simulink model "SecRwLtStCalib"  (R2024b)
settings: Solver=FixedStepDiscrete  StartTime=0.0  StopTime=10.0  FixedStep=0.01  RelTol=1e-3
model workspace (MAT data in the model file):
  KeSMSwAcsMd6SecRwLtStBkReclnUpwdDnwdPos1Max_Val : Simulink.Parameter (value not decoded)
  KeSMSwAcsMd6SecRwLtStBkReclnUpwdDnwdPos1Min_Val : Simulink.Parameter (value not decoded)
  KeSMSwAcsMd6SecRwLtStBkReclnUpwdDnwdPos1_Val : Simulink.Parameter (value not decoded)
  KeSMSwAcsMd6SecRwLtStBkReclnUpwdDnwdPosMax_Val : Simulink.Parameter (value not decoded)
  KeSMSwAcsMd6SecRwLtStBkReclnUpwdDnwdPosMin_Val : Simulink.Parameter (value not decoded)
  KeSMSwAcsMd6SecRwLtStBkReclnUpwdDnwdPos_Val : Simulink.Parameter (value not decoded)
symbols that are objects in the model workspace (value not decoded): KeSMSwAcsMd6SecRwLtStBkReclnUpwdDnwdPos1_Val, KeSMSwAcsMd6SecRwLtStBkReclnUpwdDnwdPos1Max_Val, KeSMSwAcsMd6SecRwLtStBkReclnUpwdDnwdPos1Min_Val, KeSMSwAcsMd6SecRwLtStBkReclnUpwdDnwdPos_Val, KeSMSwAcsMd6SecRwLtStBkReclnUpwdDnwdPosMax_Val, KeSMSwAcsMd6SecRwLtStBkReclnUpwdDnwdPosMin_Val
undefined symbols (not defined in the file or in its folder): KeSMSw4SAcsMd21SecRwLtStBkReclnUpwdDnwdPos_Val, KeSMSw4SAcsMd21SecRwLtStBkReclnUpwdDnwdPosMax_Val, KeSMSw4SAcsMd21SecRwLtStBkReclnUpwdDnwdPosMin_Val, KeSMSw4SAcsMd21SecRwLtStFrwdBkwdPos_Val, KeSMSw4SAcsMd21SecRwLtStFrwdBkwdPosMax_Val, KeSMSw4SAcsMd21SecRwLtStFrwdBkwdPosMin_Val, KeSMSw4SAcsMd21SecRwLtStHdrstFrwdBkwdPos_Val, KeSMSw4SAcsMd21SecRwLtStHdrstFrwdBkwdPosMax_Val, KeSMSw4SAcsMd21SecRwLtStHdrstFrwdBkwdPosMin_Val, KeSMSw4SAcsMd21SecRwLtStHdrstUpwdDnwdPos_Val, KeSMSw4SAcsMd21SecRwLtStHdrstUpwdDnwdPosMax_Val, KeSMSw4SAcsMd21SecRwLtStHdrstUpwdDnwdPosMin_Val, KeSMSw4SAcsMd22SecRwLtStBkReclnUpwdDnwdPos1_Val, KeSMSw4SAcsMd22SecRwLtStBkReclnUpwdDnwdPos2_Val, KeSMSw4SAcsMd22SecRwLtStBkReclnUpwdDnwdPos2Max_Val, KeSMSw4SAcsMd22SecRwLtStBkReclnUpwdDnwdPos2Min_Val, KeSMSw4SAcsMd22SecRwLtStBkReclnUpwdDnwdPosMax_Val, KeSMSw4SAcsMd22SecRwLtStBkReclnUpwdDnwdPosMin_Val, KeSMSw4SAcsMd22SecRwLtStFrwdBkwdPos_Val, KeSMSw4SAcsMd22SecRwLtStFrwdBkwdPosMax_Val, KeSMSw4SAcsMd22SecRwLtStFrwdBkwdPosMin_Val, KeSMSw4SAcsMd22SecRwLtStFtrstUpwdDnwdPos_Val, KeSMSw4SAcsMd22SecRwLtStFtrstUpwdDnwdPosMax_Val, KeSMSw4SAcsMd22SecRwLtStFtrstUpwdDnwdPosMin_Val, KeSMSw4SAcsMd22SecRwLtStHdrstFrwdBkwdPos_Val, KeSMSw4SAcsMd22SecRwLtStHdrstFrwdBkwdPosMax_Val, KeSMSw4SAcsMd22SecRwLtStHdrstFrwdBkwdPosMin_Val, KeSMSw4SAcsMd22SecRwLtStHdrstUpwdDnwdPos_Val, KeSMSw4SAcsMd22SecRwLtStHdrstUpwdDnwdPosMax_Val, KeSMSw4SAcsMd22SecRwLtStHdrstUpwdDnwdPosMin_Val, KeSMSw4SAcsMd22SecRwLtStLegrstOtwdInwdPos_Val, KeSMSw4SAcsMd22SecRwLtStLegrstOtwdInwdPosMax_Val, KeSMSw4SAcsMd22SecRwLtStLegrstOtwdInwdPosMin_Val, KeSMSw4SAcsMd22SecRwLtStLegrstUpwdDnwdPos_Val, KeSMSw4SAcsMd22SecRwLtStLegrstUpwdDnwdPosMax_Val, KeSMSw4SAcsMd22SecRwLtStLegrstUpwdDnwdPosMin_Val, KeSMSw4SAcsMd25SecRwLtStBkReclnUpwdDnwdPos_Val, KeSMSw4SAcsMd25SecRwLtStBkReclnUpwdDnwdPosMax_Val, KeSMSw4SAcsMd25SecRwLtStBkReclnUpwdDnwdPosMin_Val, KeSMSw4SAcsMd25SecRwLtStFrwdBkwdPos_Val, KeSMSw4SAcsMd25SecRwLtStFrwdBkwdPosMax_Val, KeSMSw4SAcsMd25SecRwLtStFrwdBkwdPosMin_Val, KeSMSw4SAcsMd25SecRwLtStHdrstFrwdBkwdPos_Val, KeSMSw4SAcsMd25SecRwLtStHdrstFrwdBkwdPosMax_Val, KeSMSw4SAcsMd25SecRwLtStHdrstFrwdBkwdPosMin_Val, KeSMSw4SAcsMd25SecRwLtStHdrstUpwdDnwdPos_Val, KeSMSw4SAcsMd25SecRwLtStHdrstUpwdDnwdPosMax_Val, KeSMSw4SAcsMd25SecRwLtStHdrstUpwdDnwdPosMin_Val, KeSMSw4SAcsMd26SecRwLtStBkReclnUpwdDnwdPos_Val, KeSMSw4SAcsMd26SecRwLtStBkReclnUpwdDnwdPosMax_Val, KeSMSw4SAcsMd26SecRwLtStBkReclnUpwdDnwdPosMin_Val, KeSMSw4SAcsMd26SecRwLtStFrwdBkwdPos_Val, KeSMSw4SAcsMd26SecRwLtStFrwdBkwdPosMax_Val, KeSMSw4SAcsMd26SecRwLtStFrwdBkwdPosMin_Val, KeSMSw4SAcsMd26SecRwLtStFtrstUpwdDnwdPos_Val, KeSMSw4SAcsMd26SecRwLtStFtrstUpwdDnwdPosMax_Val, KeSMSw4SAcsMd26SecRwLtStFtrstUpwdDnwdPosMin_Val, KeSMSw4SAcsMd26SecRwLtStHdrstFrwdBkwdPos_Val, KeSMSw4SAcsMd26SecRwLtStHdrstFrwdBkwdPosMax_Val, KeSMSw4SAcsMd26SecRwLtStHdrstFrwdBkwdPosMin_Val ... (+496)
libraries: TrgtPosSelcLib x61, StIsPosChkLib x1, simulink x1
(part 6 of 8)

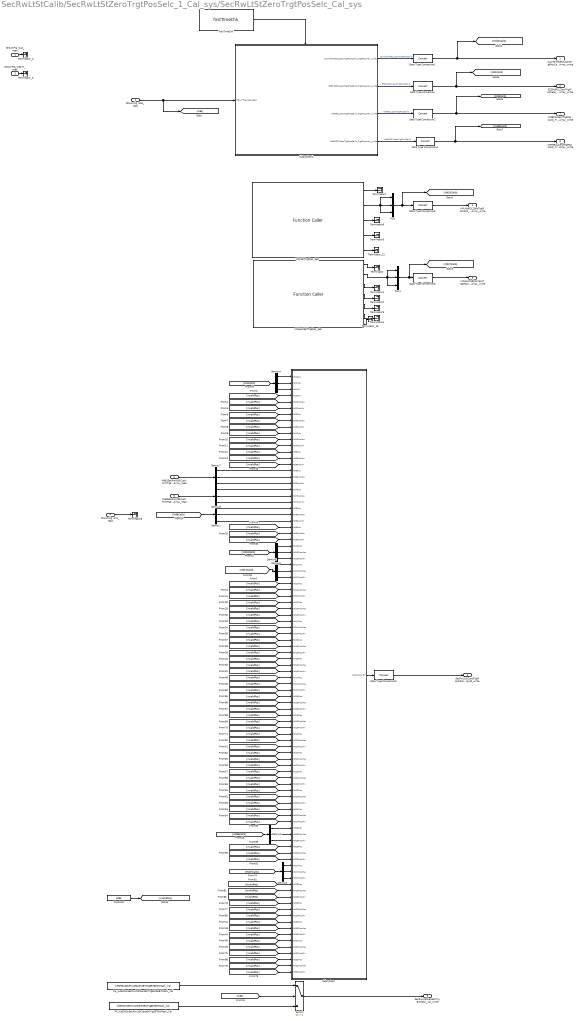
== system SecRwLtStCalib/SecRwLtStZeroTrgtPosSelc_1_Cal_sys/SecRwLtStZeroTrgtPosSelc_Cal_sys ==
  StNumFlg_Is4s_read : Inport
  StNumFlg_Is6s_read : Inport  Port=2
  StNumFlg_Is6s7s_read : Inport  Port=3
  StNumFlg_Is7s_read : Inport  Port=4
  Md61SecRwRtStCushFrntTrgtPosCalib_TrgtPosArray_read : Inport  Port=5
  Md62SecRwLtStCushFrntTrgtPosCalib_TrgtPosArray_read : Inport  Port=6
  Constant : Constant  Value=4095  OutDataTypeStr=uint16
  Data Type Conversion{,1..6} (7 alike) : DataTypeConversion  SaturateOnIntegerOverflow=off  RndMeth=Floor
  Demux{1..8} (8 alike) : Demux  Outputs=3
  Mux : Mux  Inputs=3
  Mux1 : Mux  Inputs=3
  PA_KeSMSwSecRwLtStZeroEnTrig5576sBitMask_Val : Constant  Value=KeSMSwSecRwLtStZeroEnTrig5576sBitMask_Val
  PA_KeSMSwSecRwLtStZeroEnTrig557BitMask_Val : Constant  Value=KeSMSwSecRwLtStZeroEnTrig557BitMask_Val
  Subsystem : Subsystem
  Subsystem1 : Subsystem
  Switch : Switch  Criteria=u2 > Threshold  SaturateOnIntegerOverflow=off  InputSameDT=off
  Terminator{,1..8} (9 alike) : Terminator
  Terminator_{3,5,12..13} (4 alike) : Terminator
  VIPL557TrgtPos_Get : FunctionCaller  FunctionPrototype=[SecRwLtStBkReclnTrgtPos,SecRwLtStZeroTrgtPos,SecRwLtStLgrstUpwdDnwdTrgtPos,SecRwLtStLgrstInwdOtwdTrgtPos,SecRwLtStFwdBkwdTrgtPos] = VIPL557TrgtPos_Get()  InputArgumentSpecifications=<Enter example>  OutputArgumentSpecifications=uint16(1), uint16(1), uint16(1), uint16(1), uint16(1)
  VIPLExit557TrgtPos_Get : FunctionCaller  FunctionPrototype=[SecRwLtStBkReclnTrgtPos,SecRwLtStZeroTrgtPos,SecRwLtStLgrstUpwdDnwdTrgtPos,SecRwLtStLgrstInwdOtwdTrgtPos,ThdRwLtStBkReclnTrgtPos,ThdRwLtStFwdBkwdTrgtPos,SecRwLtStFwdBkwdTrgtPos] = VIPLExit557TrgtPos_Get()  InputArgumentSpecifications=<Enter example>  OutputArgumentSpecifications=uint16(1), uint16(1), uint16(1), uint16(1), uint16(1), uint16(1), uint16(1)
  firstTimeChk : TrgtPosSelcLib/firstTimeChk  SystemSampleTime=-1  VariantActivationTime=update diagram  AllowFlexibleInterface=on  Latency=0  AutoFrameSizeCalculation=off
  ComfortMdR2LZeroTrgtPosCalib_TrgtPosArray_write : Outport  VectorParamsAs1DForOutWhenUnconnected=off
      settings: EnsureOutportIsVirtual=on
  EZEMdR2LZeroTrgtPosCalib_TrgtPosArray_write : Outport  Port=2  VectorParamsAs1DForOutWhenUnconnected=off
      settings: EnsureOutportIsVirtual=on
  SecRwLtStZeroTrgtPosCalibArray32_TrgtPosArray32_write : Outport  Port=3  VectorParamsAs1DForOutWhenUnconnected=off
      settings: EnsureOutportIsVirtual=on
  VIPLMdR2LZeroTrgtPosCalib_TrgtPosArray_write : Outport  Port=4  VectorParamsAs1DForOutWhenUnconnected=off
      settings: EnsureOutportIsVirtual=on
  VIPLExitMdR2LZeroTrgtPosCalib_TrgtPosArray_write : Outport  Port=5  VectorParamsAs1DForOutWhenUnconnected=off
      settings: EnsureOutportIsVirtual=on
  SecRwLtStZeroEnTrigBitMask_Val_write : Outport  Port=6  VectorParamsAs1DForOutWhenUnconnected=off
      settings: EnsureOutportIsVirtual=on
  Md8R2LZeroTrgtPosCalib_TrgtPosArray_write : Outport  Port=7  VectorParamsAs1DForOutWhenUnconnected=off
      settings: EnsureOutportIsVirtual=on
  Md56R2LZeroTrgtPosCalib_TrgtPosArray_write : Outport  Port=8  VectorParamsAs1DForOutWhenUnconnected=off
      settings: EnsureOutportIsVirtual=on
  wires:
  StNumFlg_Is4s_read/1 -> Terminator_3/1
  StNumFlg_Is6s7s_read/1 -> Terminator_5/1
  Mux/1 -> [Md10Calib], Data Type Conversion5/1
  VIPLExit557TrgtPos_Get/2 -> Mux1/3, Mux1/1, Mux1/2
  Mux1/1 -> [Md27Calib], Data Type Conversion6/1
  VIPLExit557TrgtPos_Get/1 -> Terminator/1
  VIPLExit557TrgtPos_Get/3 -> Terminator1/1
  VIPLExit557TrgtPos_Get/4 -> Terminator2/1
  VIPLExit557TrgtPos_Get/5 -> Terminator3/1
  VIPLExit557TrgtPos_Get/6 -> Terminator4/1
  VIPL557TrgtPos_Get/4 -> Terminator5/1
  VIPL557TrgtPos_Get/3 -> Terminator6/1
  VIPL557TrgtPos_Get/1 -> Terminator7/1
  VIPL557TrgtPos_Get/2 -> Mux/3, Mux/1, Mux/2
  Data Type Conversion3/1 -> SecRwLtStZeroTrgtPosCalibArray32_TrgtPosArray32_write/1
  Demux1/3 -> Subsystem/24(Md8PosMin)
  [invalidPos] -> Subsystem/85(Md29Pos)
  [invalidPos] -> Subsystem/10(Md4Pos)
  [invalidPos] -> Subsystem/50(Md17PosMax)
  [invalidPos] -> Subsystem/77(Md26PosMax)
  Demux1/1 -> Subsystem/22(Md8Pos)
  [invalidPos] -> Subsystem/9(Md3PosMin)
  [invalidPos] -> Subsystem/76(Md26Pos)
  [invalidPos] -> Subsystem/25(Md9Pos)
  [invalidPos] -> Subsystem/46(Md16Pos)
  [invalidPos] -> Subsystem/72(Md24PosMin)
  Demux5/3 -> Subsystem/30(Md10PosMin)
  [invalidPos] -> Subsystem/45(Md15PosMin)
  [invalidPos] -> Subsystem/63(Md21PosMin)
  [invalidPos] -> Subsystem/58(Md20Pos)
  [invalidPos] -> Subsystem/53(Md18PosMax)
  Demux4/1 -> Subsystem/1(Md1Pos)
  [invalidPos] -> Subsystem/55(Md19Pos)
  [invalidPos] -> Subsystem/86(Md29PosMax)
  [invalidPos] -> Subsystem/68(Md23PosMax)
  [invalidPos] -> Subsystem/62(Md21PosMax)
  [invalidPos] -> Subsystem/14(Md5PosMax)
  [invalidPos] -> Subsystem/87(Md29PosMin)
  Demux1/2 -> Subsystem/23(Md8PosMax)
  [invalidPos] -> Subsystem/26(Md9PosMax)
  [invalidPos] -> Subsystem/94(Md32Pos)
  [invalidPos] -> Subsystem/54(Md18PosMin)
  [invalidPos] -> Subsystem/61(Md21Pos)
  [invalidPos] -> Subsystem/5(Md2PosMax)
  [invalidPos] -> Subsystem/13(Md5Pos)
  [invalidPos] -> Subsystem/96(Md32PosMin)
  [invalidPos] -> Subsystem/59(Md20PosMax)
  [invalidPos] -> Subsystem/78(Md26PosMin)
  [invalidPos] -> Subsystem/11(Md4PosMax)
  Demux3/1 -> Subsystem/73(Md25Pos)
  [invalidPos] -> Subsystem/66(Md22PosMin)
  Demux4/2 -> Subsystem/2(Md1Max)
  [invalidPos] -> Subsystem/70(Md24Pos)
  [invalidPos] -> Subsystem/44(Md15PosMax)
  [invalidPos] -> Subsystem/60(Md20PosMin)
  [invalidPos] -> Subsystem/64(Md22Pos)
  [invalidPos] -> Subsystem/51(Md17PosMin)
  [invalidPos] -> Subsystem/43(Md15Pos)
  [invalidPos] -> Subsystem/57(Md19PosMin)
  [invalidPos] -> Subsystem/67(Md23Pos)
  [invalidPos] -> Subsystem/4(Md2Pos)
  [invalidPos] -> Subsystem/49(Md17Pos)
  [invalidPos] -> Subsystem/71(Md24PosMax)
  [invalidPos] -> Subsystem/65(Md22PosMax)
  [invalidPos] -> Subsystem/6(Md2PosMin)
  Demux3/3 -> Subsystem/75(Md25PosMin)
  [invalidPos] -> Subsystem/37(Md13Pos)
  [invalidPos] -> Subsystem/52(Md18Pos)
  Demux3/2 -> Subsystem/74(Md25PosMax)
  [invalidPos] -> Subsystem/27(Md9PosMin)
  [invalidPos] -> Subsystem/48(Md16PosMin)
  [invalidPos] -> Subsystem/41(Md14PosMax)
  Demux5/1 -> Subsystem/28(Md10Pos)
  [invalidPos] -> Subsystem/38(Md13PosMax)
  [invalidPos] -> Subsystem/47(Md16PosMax)
  [invalidPos] -> Subsystem/56(Md19PosMax)
  [invalidPos] -> Subsystem/39(Md13PosMin)
  [invalidPos] -> Subsystem/40(Md14Pos)
  Subsystem/1(CalibArray32) -> Data Type Conversion3/1
  [invalidPos] -> Subsystem/42(Md14PosMin)
  [invalidPos] -> Subsystem/12(Md4PosMin)
  [invalidPos] -> Subsystem/69(Md23PosMin)
  [invalidPos] -> Subsystem/82(Md28Pos)
  [invalidPos] -> Subsystem/15(Md5PosMin)
  Demux4/3 -> Subsystem/3(Md1Min)
  [invalidPos] -> Subsystem/95(Md32PosMax)
  [invalidPos] -> Subsystem/8(Md3PosMax)
  [invalidPos] -> Subsystem/7(Md3Pos)
  Demux5/2 -> Subsystem/29(Md10PosMax)
  [Md1Calib] -> Demux4/1
  [Md10Calib] -> Demux5/1
  Demux6/1 -> Subsystem/31(Md11Pos)
  Demux6/2 -> Subsystem/32(Md11PosMax)
  Demux6/3 -> Subsystem/33(Md11PosMin)
  [Md11Calib] -> Demux6/1
  [invalidPos] -> Subsystem/34(Md12Pos)
  [invalidPos] -> Subsystem/35(Md12PosMax)
  [invalidPos] -> Subsystem/36(Md12PosMin)
  [Md27Calib] -> Demux2/1
  Demux2/1 -> Subsystem/79(Md27Pos)
  Demux2/2 -> Subsystem/80(Md27PosMax)
  Demux2/3 -> Subsystem/81(Md27PosMin)
  [invalidPos] -> Subsystem/83(Md28PosMax)
  [invalidPos] -> Subsystem/84(Md28PosMin)
  [invalidPos] -> Subsystem/88(Md30Pos)
  [invalidPos] -> Subsystem/89(Md30PosMax)
  [invalidPos] -> Subsystem/90(Md30PosMin)
  [invalidPos] -> Subsystem/91(Md31Pos)
  [invalidPos] -> Subsystem/92(Md31PosMax)
  [invalidPos] -> Subsystem/93(Md31PosMin)
  Constant/1 -> [invalidPos]
  VIPL557TrgtPos_Get/5 -> Terminator_12/1
  VIPLExit557TrgtPos_Get/7 -> Terminator_13/1
  [Md8Calib] -> Demux1/1
  StNumFlg_Is7s_read/1 -> Terminator8/1
  Switch/1 -> SecRwLtStZeroEnTrigBitMask_Val_write/1
  [Is6s] -> Switch/2
  PA_KeSMSwSecRwLtStZeroEnTrig5576sBitMask_Val/1 -> Switch/1
  PA_KeSMSwSecRwLtStZeroEnTrig557BitMask_Val/1 -> Switch/3
  firstTimeChk/1 -> Subsystem1/Enable
  StNumFlg_Is6s_read/1 -> [Is6s], Subsystem1/1(StNumFlg_Is6s_read)
  Subsystem1/4(Md56R2LZeroTrgtPosCalib_TrgtPosArray_write) -> Data Type Conversion4/1  "Md56R2LZeroTrgtPosCalib"
  Subsystem1/1(ComfortMdR2LZeroTrgtPosCalib_TrgtPosArray_write) -> Data Type Conversion1/1  "ComfortMdR2LZeroTrgtPosCalib"
  Subsystem1/2(EZEMdR2LZeroTrgtPosCalib_TrgtPosArray_write) -> Data Type Conversion/1  "EZEMdR2LZeroTrgtPosCalib"
  Subsystem1/3(Md8R2LZeroTrgtPosCalib_TrgtPosArray_write) -> Data Type Conversion2/1  "Md8R2LZeroTrgtPosCalib"
  [Md56Calib] -> Demux3/1
  Data Type Conversion1/1 -> [Md11Calib], ComfortMdR2LZeroTrgtPosCalib_TrgtPosArray_write/1
  Data Type Conversion/1 -> [Md1Calib], EZEMdR2LZeroTrgtPosCalib_TrgtPosArray_write/1
  Data Type Conversion2/1 -> [Md8Calib], Md8R2LZeroTrgtPosCalib_TrgtPosArray_write/1
  Data Type Conversion4/1 -> [Md56Calib], Md56R2LZeroTrgtPosCalib_TrgtPosArray_write/1
  Data Type Conversion5/1 -> VIPLMdR2LZeroTrgtPosCalib_TrgtPosArray_write/1
  Data Type Conversion6/1 -> VIPLExitMdR2LZeroTrgtPosCalib_TrgtPosArray_write/1
  Demux7/1 -> Subsystem/16(Md6Pos)
  Demux7/2 -> Subsystem/17(Md6PosMax)
  Demux7/3 -> Subsystem/18(Md6PosMin)
  Md61SecRwRtStCushFrntTrgtPosCalib_TrgtPosArray_read/1 -> Demux7/1
  Demux8/1 -> Subsystem/19(Md7Pos)
  Demux8/2 -> Subsystem/20(Md7PosMax)
  Demux8/3 -> Subsystem/21(Md7PosMin)
  Md62SecRwLtStCushFrntTrgtPosCalib_TrgtPosArray_read/1 -> Demux8/1

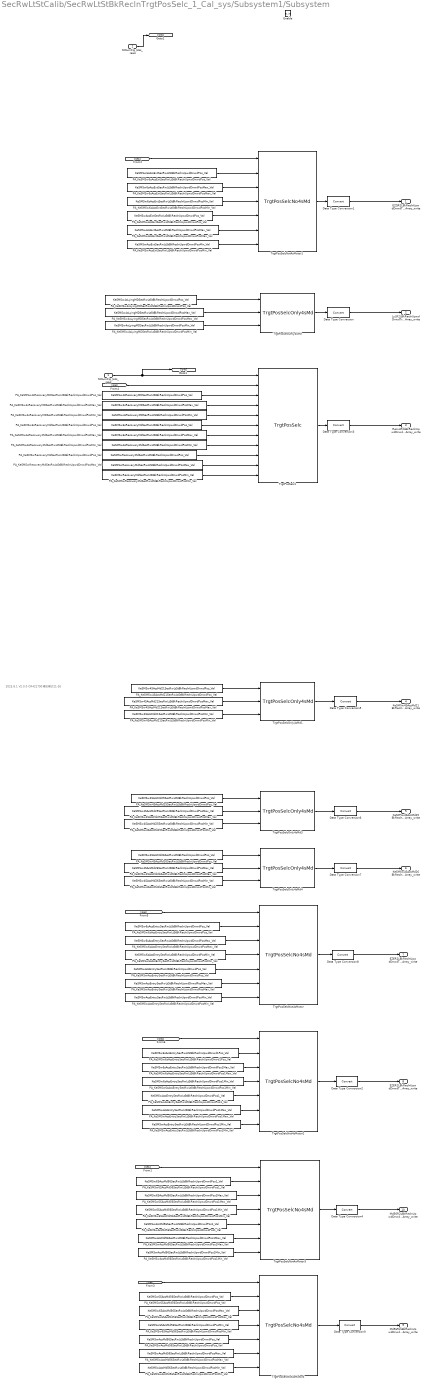
== system SecRwLtStCalib/SecRwLtStBkReclnTrgtPosSelc_1_Cal_sys/Subsystem1/Subsystem ==
  note: 2023.8.1 V2.0.0 CR421790 增加模式21-26
  StNumFlg_Is4s_read : Inport
  StNumFlg_Is6s_read : Inport  Port=2
  Enable : EnablePort
  Data Type Conversion{,1..9} (10 alike) : DataTypeConversion  SaturateOnIntegerOverflow=off  RndMeth=Floor
  PA_KeSMSw4SAcsMd21SecRwLtStBkReclnUpwdDnwdPosMax_Val : Constant  Value=KeSMSw4SAcsMd21SecRwLtStBkReclnUpwdDnwdPosMax_Val
  PA_KeSMSw4SAcsMd21SecRwLtStBkReclnUpwdDnwdPosMin_Val : Constant  Value=KeSMSw4SAcsMd21SecRwLtStBkReclnUpwdDnwdPosMin_Val
  PA_KeSMSw4SAcsMd21SecRwLtStBkReclnUpwdDnwdPos_Val : Constant  Value=KeSMSw4SAcsMd21SecRwLtStBkReclnUpwdDnwdPos_Val
  PA_KeSMSw4SAcsMd25SecRwLtStBkReclnUpwdDnwdPosMax_Val : Constant  Value=KeSMSw4SAcsMd25SecRwLtStBkReclnUpwdDnwdPosMax_Val
  PA_KeSMSw4SAcsMd25SecRwLtStBkReclnUpwdDnwdPosMin_Val : Constant  Value=KeSMSw4SAcsMd25SecRwLtStBkReclnUpwdDnwdPosMin_Val
  PA_KeSMSw4SAcsMd25SecRwLtStBkReclnUpwdDnwdPos_Val : Constant  Value=KeSMSw4SAcsMd25SecRwLtStBkReclnUpwdDnwdPos_Val
  PA_KeSMSw4SAcsMd26SecRwLtStBkReclnUpwdDnwdPosMax_Val : Constant  Value=KeSMSw4SAcsMd26SecRwLtStBkReclnUpwdDnwdPosMax_Val
  PA_KeSMSw4SAcsMd26SecRwLtStBkReclnUpwdDnwdPosMin_Val : Constant  Value=KeSMSw4SAcsMd26SecRwLtStBkReclnUpwdDnwdPosMin_Val
  PA_KeSMSw4SAcsMd26SecRwLtStBkReclnUpwdDnwdPos_Val : Constant  Value=KeSMSw4SAcsMd26SecRwLtStBkReclnUpwdDnwdPos_Val
  PA_KeSMSw4sLyingMDSecRwLtStBkReclnUpwdDnwdPosMax_Val : Constant  Value=KeSMSw4sLyingMDSecRwLtStBkReclnUpwdDnwdPosMax_Val
  PA_KeSMSw4sLyingMDSecRwLtStBkReclnUpwdDnwdPosMin_Val : Constant  Value=KeSMSw4sLyingMDSecRwLtStBkReclnUpwdDnwdPosMin_Val
  PA_KeSMSw4sLyingMDSecRwLtStBkReclnUpwdDnwdPos_Val : Constant  Value=KeSMSw4sLyingMDSecRwLtStBkReclnUpwdDnwdPos_Val
  PA_KeSMSw4sRecoveryMDSecRwLtStBkReclnUpwdDnwdPosMax_Val : Constant  Value=KeSMSw4sRecoveryMDSecRwLtStBkReclnUpwdDnwdPosMax_Val
  PA_KeSMSw4sRecoveryMDSecRwLtStBkReclnUpwdDnwdPosMin_Val : Constant  Value=KeSMSw4sRecoveryMDSecRwLtStBkReclnUpwdDnwdPosMin_Val
  PA_KeSMSw4sRecoveryMDSecRwLtStBkReclnUpwdDnwdPos_Val : Constant  Value=KeSMSw4sRecoveryMDSecRwLtStBkReclnUpwdDnwdPos_Val
  PA_KeSMSw6SAcsMd56SecRwLtStBkReclnUpwdDnwdPos1Max_Val : Constant  Value=KeSMSw6SAcsMd56SecRwLtStBkReclnUpwdDnwdPos1Max_Val
  PA_KeSMSw6SAcsMd56SecRwLtStBkReclnUpwdDnwdPos1Min_Val : Constant  Value=KeSMSw6SAcsMd56SecRwLtStBkReclnUpwdDnwdPos1Min_Val
  PA_KeSMSw6SAcsMd56SecRwLtStBkReclnUpwdDnwdPos1_Val : Constant  Value=KeSMSw6SAcsMd56SecRwLtStBkReclnUpwdDnwdPos1_Val
  PA_KeSMSw6SAcsMd56SecRwLtStBkReclnUpwdDnwdPosMax_Val : Constant  Value=KeSMSw6SAcsMd56SecRwLtStBkReclnUpwdDnwdPosMax_Val
  PA_KeSMSw6SAcsMd56SecRwLtStBkReclnUpwdDnwdPosMin_Val : Constant  Value=KeSMSw6SAcsMd56SecRwLtStBkReclnUpwdDnwdPosMin_Val
  PA_KeSMSw6SAcsMd56SecRwLtStBkReclnUpwdDnwdPos_Val : Constant  Value=KeSMSw6SAcsMd56SecRwLtStBkReclnUpwdDnwdPos_Val
  PA_KeSMSw6sAcsEntrySecRwLtStBkReclnUpwdDnwd1Pos_Val : Constant  Value=KeSMSw6sAcsEntrySecRwLtStBkReclnUpwdDnwd1Pos_Val
  PA_KeSMSw6sAcsEntrySecRwLtStBkReclnUpwdDnwdPos1Max_Val : Constant  Value=KeSMSw6sAcsEntrySecRwLtStBkReclnUpwdDnwdPos1Max_Val
  PA_KeSMSw6sAcsEntrySecRwLtStBkReclnUpwdDnwdPos1Min_Val : Constant  Value=KeSMSw6sAcsEntrySecRwLtStBkReclnUpwdDnwdPos1Min_Val
  PA_KeSMSw6sAcsEntrySecRwLtStBkReclnUpwdDnwdPosMax_Val : Constant  Value=KeSMSw6sAcsEntrySecRwLtStBkReclnUpwdDnwdPosMax_Val
  PA_KeSMSw6sAcsEntrySecRwLtStBkReclnUpwdDnwdPosMin_Val : Constant  Value=KeSMSw6sAcsEntrySecRwLtStBkReclnUpwdDnwdPosMin_Val
  PA_KeSMSw6sAcsEntrySecRwLtStBkReclnUpwdDnwdPos_Val : Constant  Value=KeSMSw6sAcsEntrySecRwLtStBkReclnUpwdDnwdPos_Val
  PA_KeSMSw6sAcsExtSecRwLtStBkReclnUpwdDnwdPosMax_Val : Constant  Value=KeSMSw6sAcsExtSecRwLtStBkReclnUpwdDnwdPosMax_Val
  PA_KeSMSw6sAcsExtSecRwLtStBkReclnUpwdDnwdPosMin_Val : Constant  Value=KeSMSw6sAcsExtSecRwLtStBkReclnUpwdDnwdPosMin_Val
  PA_KeSMSw6sAcsExtSecRwLtStBkReclnUpwdDnwdPos_Val : Constant  Value=KeSMSw6sAcsExtSecRwLtStBkReclnUpwdDnwdPos_Val
  PA_KeSMSw6sRecoveryMdSecRwLtStBkReclnUpwdDnwdPosMax_Val : Constant  Value=KeSMSw6sRecoveryMdSecRwLtStBkReclnUpwdDnwdPosMax_Val
  PA_KeSMSw6sRecoveryMdSecRwLtStBkReclnUpwdDnwdPosMin_Val : Constant  Value=KeSMSw6sRecoveryMdSecRwLtStBkReclnUpwdDnwdPosMin_Val
  PA_KeSMSw6sRecoveryMdSecRwLtStBkReclnUpwdDnwdPos_Val : Constant  Value=KeSMSw6sRecoveryMdSecRwLtStBkReclnUpwdDnwdPos_Val
  PA_KeSMSwAcsEntrySecRwLtStBkReclnUpwdDnwdPos1Max_Val : Constant  Value=KeSMSwAcsEntrySecRwLtStBkReclnUpwdDnwdPos1Max_Val
  PA_KeSMSwAcsEntrySecRwLtStBkReclnUpwdDnwdPos1Min_Val : Constant  Value=KeSMSwAcsEntrySecRwLtStBkReclnUpwdDnwdPos1Min_Val
  PA_KeSMSwAcsEntrySecRwLtStBkReclnUpwdDnwdPos1_Val : Constant  Value=KeSMSwAcsEntrySecRwLtStBkReclnUpwdDnwdPos1_Val
  PA_KeSMSwAcsEntrySecRwLtStBkReclnUpwdDnwdPosMax_Val : Constant  Value=KeSMSwAcsEntrySecRwLtStBkReclnUpwdDnwdPosMax_Val
  PA_KeSMSwAcsEntrySecRwLtStBkReclnUpwdDnwdPosMin_Val : Constant  Value=KeSMSwAcsEntrySecRwLtStBkReclnUpwdDnwdPosMin_Val
  PA_KeSMSwAcsEntrySecRwLtStBkReclnUpwdDnwdPos_Val : Constant  Value=KeSMSwAcsEntrySecRwLtStBkReclnUpwdDnwdPos_Val
  PA_KeSMSwAcsExtSecRwLtStBkReclnUpwdDnwdPosMax_Val : Constant  Value=KeSMSwAcsExtSecRwLtStBkReclnUpwdDnwdPosMax_Val
  PA_KeSMSwAcsExtSecRwLtStBkReclnUpwdDnwdPosMin_Val : Constant  Value=KeSMSwAcsExtSecRwLtStBkReclnUpwdDnwdPosMin_Val
  PA_KeSMSwAcsExtSecRwLtStBkReclnUpwdDnwdPos_Val : Constant  Value=KeSMSwAcsExtSecRwLtStBkReclnUpwdDnwdPos_Val
  PA_KeSMSwAcsMd56SecRwLtStBkReclnUpwdDnwdPos1Max_Val : Constant  Value=KeSMSwAcsMd56SecRwLtStBkReclnUpwdDnwdPos1Max_Val
  PA_KeSMSwAcsMd56SecRwLtStBkReclnUpwdDnwdPos1Min_Val : Constant  Value=KeSMSwAcsMd56SecRwLtStBkReclnUpwdDnwdPos1Min_Val
  PA_KeSMSwAcsMd56SecRwLtStBkReclnUpwdDnwdPos1_Val : Constant  Value=KeSMSwAcsMd56SecRwLtStBkReclnUpwdDnwdPos1_Val
  PA_KeSMSwAcsMd56SecRwLtStBkReclnUpwdDnwdPosMax_Val : Constant  Value=KeSMSwAcsMd56SecRwLtStBkReclnUpwdDnwdPosMax_Val
  PA_KeSMSwAcsMd56SecRwLtStBkReclnUpwdDnwdPosMin_Val : Constant  Value=KeSMSwAcsMd56SecRwLtStBkReclnUpwdDnwdPosMin_Val
  PA_KeSMSwAcsMd56SecRwLtStBkReclnUpwdDnwdPos_Val : Constant  Value=KeSMSwAcsMd56SecRwLtStBkReclnUpwdDnwdPos_Val
  PA_KeSMSwRecoveryMdSecRwLtStBkReclnUpwdDnwdPosMax_Val : Constant  Value=KeSMSwRecoveryMdSecRwLtStBkReclnUpwdDnwdPosMax_Val
  PA_KeSMSwRecoveryMdSecRwLtStBkReclnUpwdDnwdPosMin_Val : Constant  Value=KeSMSwRecoveryMdSecRwLtStBkReclnUpwdDnwdPosMin_Val
  PA_KeSMSwRecoveryMdSecRwLtStBkReclnUpwdDnwdPos_Val : Constant  Value=KeSMSwRecoveryMdSecRwLtStBkReclnUpwdDnwdPos_Val
  TrgtPosSelc1 : TrgtPosSelcLib/TrgtPosSelc  SystemSampleTime=-1  VariantActivationTime=update diagram  AllowFlexibleInterface=on  Latency=0  AutoFrameSizeCalculation=off
  TrgtPosSelcNot4sMotor{,1..4} (5 alike) : TrgtPosSelcLib/TrgtPosSelcNo4sMd  SystemSampleTime=-1  VariantActivationTime=update diagram  AllowFlexibleInterface=on  Latency=0  AutoFrameSizeCalculation=off
  TrgtPosSelcOnly4sMd{,1,3..4} (4 alike) : TrgtPosSelcLib/TrgtPosSelcOnly4sMd  SystemSampleTime=-1  VariantActivationTime=update diagram  AllowFlexibleInterface=on  Latency=0  AutoFrameSizeCalculation=off
  EZQR2LBkReclnUpwdDnwdTrgtPosCalib_TrgtPosArray_write : Outport  VectorParamsAs1DForOutWhenUnconnected=off
      settings: EnsureOutportIsVirtual=on
  LyLR2LBkReclnUpwdDnwdTrgtPosCalib_TrgtPosArray_write : Outport  Port=2  VectorParamsAs1DForOutWhenUnconnected=off
  RecvLR2LBkReclnUpwdDnwdTrgtPosCalib_TrgtPosArray_write : Outport  Port=3  VectorParamsAs1DForOutWhenUnconnected=off
      settings: EnsureOutportIsVirtual=on
  KeSMSw4SAcsMd21BkReclnUpwdDnwdTrgtPosCalib_TrgtPosArray_write : Outport  Port=4  InitialOutput=0  VectorParamsAs1DForOutWhenUnconnected=off
  KeSMSw4SAcsMd25BkReclnUpwdDnwdTrgtPosCalib_TrgtPosArray_write : Outport  Port=5  InitialOutput=0  VectorParamsAs1DForOutWhenUnconnected=off
  KeSMSw4SAcsMd26BkReclnUpwdDnwdTrgtPosCalib_TrgtPosArray_write : Outport  Port=6  InitialOutput=0  VectorParamsAs1DForOutWhenUnconnected=off
  EZER2LBkReclnUpwdDnwdTrgtPosCalib_TrgtPosArray_write : Outport  Port=7  VectorParamsAs1DForOutWhenUnconnected=off
  EZER2LBkReclnUpwdDnwdTrgtPosCalib1_TrgtPosArray_write : Outport  Port=8  VectorParamsAs1DForOutWhenUnconnected=off
  Md56R2LBkReclnUpwdDnwdTrgtPosCalib_TrgtPosArray_write : Outport  Port=9  VectorParamsAs1DForOutWhenUnconnected=off
      settings: EnsureOutportIsVirtual=on
  Md56R2LBkReclnUpwdDnwdTrgtPosCalib1_TrgtPosArray_write : Outport  Port=10  VectorParamsAs1DForOutWhenUnconnected=off
      settings: EnsureOutportIsVirtual=on
  wires:
  [is6s] -> TrgtPosSelcNot4sMotor1/1
  PA_KeSMSw4sLyingMDSecRwLtStBkReclnUpwdDnwdPosMax_Val/1 -> TrgtPosSelcOnly4sMd/2
  PA_KeSMSwAcsExtSecRwLtStBkReclnUpwdDnwdPosMin_Val/1 -> TrgtPosSelcNot4sMotor1/7
  PA_KeSMSw4sLyingMDSecRwLtStBkReclnUpwdDnwdPos_Val/1 -> TrgtPosSelcOnly4sMd/1
  TrgtPosSelcOnly4sMd/1 -> Data Type Conversion/1
  StNumFlg_Is4s_read/1 -> [is4s], TrgtPosSelc1/1
  PA_KeSMSw6sAcsExtSecRwLtStBkReclnUpwdDnwdPos_Val/1 -> TrgtPosSelcNot4sMotor1/2
  PA_KeSMSw4sRecoveryMDSecRwLtStBkReclnUpwdDnwdPosMax_Val/1 -> TrgtPosSelc1/4
  PA_KeSMSw4sLyingMDSecRwLtStBkReclnUpwdDnwdPosMin_Val/1 -> TrgtPosSelcOnly4sMd/3
  PA_KeSMSw4sRecoveryMDSecRwLtStBkReclnUpwdDnwdPos_Val/1 -> TrgtPosSelc1/3
  PA_KeSMSw6sAcsExtSecRwLtStBkReclnUpwdDnwdPosMin_Val/1 -> TrgtPosSelcNot4sMotor1/4
  StNumFlg_Is6s_read/1 -> [is6s]
  PA_KeSMSwAcsExtSecRwLtStBkReclnUpwdDnwdPosMax_Val/1 -> TrgtPosSelcNot4sMotor1/6
  PA_KeSMSw6sAcsExtSecRwLtStBkReclnUpwdDnwdPosMax_Val/1 -> TrgtPosSelcNot4sMotor1/3
  PA_KeSMSw6sRecoveryMdSecRwLtStBkReclnUpwdDnwdPos_Val/1 -> TrgtPosSelc1/6
  PA_KeSMSw6sRecoveryMdSecRwLtStBkReclnUpwdDnwdPosMin_Val/1 -> TrgtPosSelc1/8
  PA_KeSMSwRecoveryMdSecRwLtStBkReclnUpwdDnwdPosMax_Val/1 -> TrgtPosSelc1/10
  TrgtPosSelc1/1 -> Data Type Conversion3/1
  TrgtPosSelcNot4sMotor1/1 -> Data Type Conversion1/1
  [is6s] -> TrgtPosSelc1/2
  PA_KeSMSwAcsExtSecRwLtStBkReclnUpwdDnwdPos_Val/1 -> TrgtPosSelcNot4sMotor1/5
  PA_KeSMSwRecoveryMdSecRwLtStBkReclnUpwdDnwdPosMin_Val/1 -> TrgtPosSelc1/11
  PA_KeSMSw6sRecoveryMdSecRwLtStBkReclnUpwdDnwdPosMax_Val/1 -> TrgtPosSelc1/7
  PA_KeSMSw4sRecoveryMDSecRwLtStBkReclnUpwdDnwdPosMin_Val/1 -> TrgtPosSelc1/5
  PA_KeSMSwRecoveryMdSecRwLtStBkReclnUpwdDnwdPos_Val/1 -> TrgtPosSelc1/9
  Data Type Conversion/1 -> LyLR2LBkReclnUpwdDnwdTrgtPosCalib_TrgtPosArray_write/1
  TrgtPosSelcOnly4sMd1/1 -> Data Type Conversion5/1
  TrgtPosSelcOnly4sMd3/1 -> Data Type Conversion6/1
  TrgtPosSelcOnly4sMd4/1 -> Data Type Conversion7/1
  PA_KeSMSw4SAcsMd21SecRwLtStBkReclnUpwdDnwdPosMin_Val/1 -> TrgtPosSelcOnly4sMd1/3
  PA_KeSMSw4SAcsMd21SecRwLtStBkReclnUpwdDnwdPosMax_Val/1 -> TrgtPosSelcOnly4sMd1/2
  PA_KeSMSw4SAcsMd21SecRwLtStBkReclnUpwdDnwdPos_Val/1 -> TrgtPosSelcOnly4sMd1/1
  PA_KeSMSw4SAcsMd26SecRwLtStBkReclnUpwdDnwdPos_Val/1 -> TrgtPosSelcOnly4sMd4/1
  PA_KeSMSw4SAcsMd26SecRwLtStBkReclnUpwdDnwdPosMax_Val/1 -> TrgtPosSelcOnly4sMd4/2
  PA_KeSMSw4SAcsMd26SecRwLtStBkReclnUpwdDnwdPosMin_Val/1 -> TrgtPosSelcOnly4sMd4/3
  PA_KeSMSw4SAcsMd25SecRwLtStBkReclnUpwdDnwdPos_Val/1 -> TrgtPosSelcOnly4sMd3/1
  PA_KeSMSw4SAcsMd25SecRwLtStBkReclnUpwdDnwdPosMax_Val/1 -> TrgtPosSelcOnly4sMd3/2
  PA_KeSMSw4SAcsMd25SecRwLtStBkReclnUpwdDnwdPosMin_Val/1 -> TrgtPosSelcOnly4sMd3/3
  Data Type Conversion1/1 -> EZQR2LBkReclnUpwdDnwdTrgtPosCalib_TrgtPosArray_write/1
  Data Type Conversion3/1 -> RecvLR2LBkReclnUpwdDnwdTrgtPosCalib_TrgtPosArray_write/1
  Data Type Conversion5/1 -> KeSMSw4SAcsMd21BkReclnUpwdDnwdTrgtPosCalib_TrgtPosArray_write/1
  Data Type Conversion6/1 -> KeSMSw4SAcsMd25BkReclnUpwdDnwdTrgtPosCalib_TrgtPosArray_write/1
  Data Type Conversion7/1 -> KeSMSw4SAcsMd26BkReclnUpwdDnwdTrgtPosCalib_TrgtPosArray_write/1
  Data Type Conversion8/1 -> EZER2LBkReclnUpwdDnwdTrgtPosCalib_TrgtPosArray_write/1
  [is6s] -> TrgtPosSelcNot4sMotor2/1
  PA_KeSMSw6sAcsEntrySecRwLtStBkReclnUpwdDnwdPos1Min_Val/1 -> TrgtPosSelcNot4sMotor2/4
  PA_KeSMSwAcsEntrySecRwLtStBkReclnUpwdDnwdPos1Min_Val/1 -> TrgtPosSelcNot4sMotor2/7
  PA_KeSMSwAcsEntrySecRwLtStBkReclnUpwdDnwdPos1_Val/1 -> TrgtPosSelcNot4sMotor2/5
  PA_KeSMSw6sAcsEntrySecRwLtStBkReclnUpwdDnwd1Pos_Val/1 -> TrgtPosSelcNot4sMotor2/2
  PA_KeSMSwAcsEntrySecRwLtStBkReclnUpwdDnwdPos1Max_Val/1 -> TrgtPosSelcNot4sMotor2/6
  [is6s] -> TrgtPosSelcNot4sMotor/1
  TrgtPosSelcNot4sMotor/1 -> Data Type Conversion8/1
  PA_KeSMSw6sAcsEntrySecRwLtStBkReclnUpwdDnwdPos1Max_Val/1 -> TrgtPosSelcNot4sMotor2/3
  PA_KeSMSwAcsEntrySecRwLtStBkReclnUpwdDnwdPosMax_Val/1 -> TrgtPosSelcNot4sMotor/6
  PA_KeSMSw6sAcsEntrySecRwLtStBkReclnUpwdDnwdPosMin_Val/1 -> TrgtPosSelcNot4sMotor/4
  PA_KeSMSwAcsEntrySecRwLtStBkReclnUpwdDnwdPos_Val/1 -> TrgtPosSelcNot4sMotor/5
  PA_KeSMSwAcsEntrySecRwLtStBkReclnUpwdDnwdPosMin_Val/1 -> TrgtPosSelcNot4sMotor/7
  PA_KeSMSw6sAcsEntrySecRwLtStBkReclnUpwdDnwdPosMax_Val/1 -> TrgtPosSelcNot4sMotor/3
  TrgtPosSelcNot4sMotor2/1 -> Data Type Conversion2/1
  PA_KeSMSw6sAcsEntrySecRwLtStBkReclnUpwdDnwdPos_Val/1 -> TrgtPosSelcNot4sMotor/2
  Data Type Conversion2/1 -> EZER2LBkReclnUpwdDnwdTrgtPosCalib1_TrgtPosArray_write/1
  PA_KeSMSw6SAcsMd56SecRwLtStBkReclnUpwdDnwdPos1Min_Val/1 -> TrgtPosSelcNot4sMotor3/4
  PA_KeSMSwAcsMd56SecRwLtStBkReclnUpwdDnwdPos1Min_Val/1 -> TrgtPosSelcNot4sMotor3/7
  PA_KeSMSwAcsMd56SecRwLtStBkReclnUpwdDnwdPos1_Val/1 -> TrgtPosSelcNot4sMotor3/5
  PA_KeSMSwAcsMd56SecRwLtStBkReclnUpwdDnwdPos1Max_Val/1 -> TrgtPosSelcNot4sMotor3/6
  PA_KeSMSw6SAcsMd56SecRwLtStBkReclnUpwdDnwdPos1_Val/1 -> TrgtPosSelcNot4sMotor3/2
  PA_KeSMSw6SAcsMd56SecRwLtStBkReclnUpwdDnwdPos1Max_Val/1 -> TrgtPosSelcNot4sMotor3/3
  [is6s] -> TrgtPosSelcNot4sMotor3/1
  TrgtPosSelcNot4sMotor3/1 -> Data Type Conversion4/1
  Data Type Conversion4/1 -> Md56R2LBkReclnUpwdDnwdTrgtPosCalib1_TrgtPosArray_write/1
  TrgtPosSelcNot4sMotor4/1 -> Data Type Conversion9/1
  Data Type Conversion9/1 -> Md56R2LBkReclnUpwdDnwdTrgtPosCalib_TrgtPosArray_write/1
  [is6s] -> TrgtPosSelcNot4sMotor4/1
  PA_KeSMSw6SAcsMd56SecRwLtStBkReclnUpwdDnwdPos_Val/1 -> TrgtPosSelcNot4sMotor4/2
  PA_KeSMSw6SAcsMd56SecRwLtStBkReclnUpwdDnwdPosMax_Val/1 -> TrgtPosSelcNot4sMotor4/3
  PA_KeSMSw6SAcsMd56SecRwLtStBkReclnUpwdDnwdPosMin_Val/1 -> TrgtPosSelcNot4sMotor4/4
  PA_KeSMSwAcsMd56SecRwLtStBkReclnUpwdDnwdPos_Val/1 -> TrgtPosSelcNot4sMotor4/5
  PA_KeSMSwAcsMd56SecRwLtStBkReclnUpwdDnwdPosMax_Val/1 -> TrgtPosSelcNot4sMotor4/6
  PA_KeSMSwAcsMd56SecRwLtStBkReclnUpwdDnwdPosMin_Val/1 -> TrgtPosSelcNot4sMotor4/7

== system SecRwLtStCalib/SecRwLtStBkReclnTrgtPosSelc_1_Cal_sys/Subsystem1/Subsystem1 ==
  note: 2023.11.7 V2.3.0 bug 554442 md22 标定分为两套
  R2LMdSeatOccupied_Val_read : Inport
  Enable : EnablePort
  Data Type Conversion : DataTypeConversion  SaturateOnIntegerOverflow=off  RndMeth=Floor
  Demux : Demux  Outputs=3
  Mux : Mux  Inputs=3
  Mux1 : Mux  Inputs=3
  PA_KeSMSw4SAcsMd22SecRwLtStBkReclnUpwdDnwdPos1Max_Val : Constant  Value=KeSMSw4SAcsMd22SecRwLtStBkReclnUpwdDnwdPosMax_Val
  PA_KeSMSw4SAcsMd22SecRwLtStBkReclnUpwdDnwdPos1Min_Val : Constant  Value=KeSMSw4SAcsMd22SecRwLtStBkReclnUpwdDnwdPosMin_Val
  PA_KeSMSw4SAcsMd22SecRwLtStBkReclnUpwdDnwdPos2Max_Val : Constant  Value=KeSMSw4SAcsMd22SecRwLtStBkReclnUpwdDnwdPos2Max_Val
  PA_KeSMSw4SAcsMd22SecRwLtStBkReclnUpwdDnwdPos2Min_Val : Constant  Value=KeSMSw4SAcsMd22SecRwLtStBkReclnUpwdDnwdPos2Min_Val
  PA_KeSMSw4SAcsMd22SecRwLtStBkReclnUpwdDnwdPos2_Val : Constant  Value=KeSMSw4SAcsMd22SecRwLtStBkReclnUpwdDnwdPos2_Val
  PA_KeSMSw4SAcsMd22SecRwLtStBkReclnUpwdDnwdPos_Val : Constant  Value=KeSMSw4SAcsMd22SecRwLtStBkReclnUpwdDnwdPos1_Val
  Switch : Switch  Criteria=u2 > Threshold  SaturateOnIntegerOverflow=off  InputSameDT=off
  TrgtPosSelcOnly4sMd2 : TrgtPosSelcLib/TrgtPosSelcOnly4sMd  SystemSampleTime=-1  VariantActivationTime=update diagram  AllowFlexibleInterface=on  Latency=0  AutoFrameSizeCalculation=off
  KeSMSw4SAcsMd22BkReclnUpwdDnwdTrgtPosCalib_TrgtPosArray_write : Outport  InitialOutput=0  VectorParamsAs1DForOutWhenUnconnected=off
  wires:
  TrgtPosSelcOnly4sMd2/1 -> Data Type Conversion/1
  R2LMdSeatOccupied_Val_read/1 -> Switch/2
  Data Type Conversion/1 -> KeSMSw4SAcsMd22BkReclnUpwdDnwdTrgtPosCalib_TrgtPosArray_write/1
  PA_KeSMSw4SAcsMd22SecRwLtStBkReclnUpwdDnwdPos2Min_Val/1 -> Mux/3
  PA_KeSMSw4SAcsMd22SecRwLtStBkReclnUpwdDnwdPos2Max_Val/1 -> Mux/2
  PA_KeSMSw4SAcsMd22SecRwLtStBkReclnUpwdDnwdPos2_Val/1 -> Mux/1
  Mux/1 -> Switch/1
  PA_KeSMSw4SAcsMd22SecRwLtStBkReclnUpwdDnwdPos1Min_Val/1 -> Mux1/3
  PA_KeSMSw4SAcsMd22SecRwLtStBkReclnUpwdDnwdPos1Max_Val/1 -> Mux1/2
  PA_KeSMSw4SAcsMd22SecRwLtStBkReclnUpwdDnwdPos_Val/1 -> Mux1/1
  Mux1/1 -> Switch/3
  Switch/1 -> Demux/1
  Demux/2 -> TrgtPosSelcOnly4sMd2/2
  Demux/1 -> TrgtPosSelcOnly4sMd2/1
  Demux/3 -> TrgtPosSelcOnly4sMd2/3

== system SecRwLtStCalib/SecRwLtStBkReclnTrgtPosSelc_1_Cal_sys/Subsystem1/Subsystem2 ==
  FirstStepPassFlg : Inport
  Cal2 : Inport  Port=2
  Cal1 : Inport  Port=3
  Switch : Switch  Criteria=u2 > Threshold  SaturateOnIntegerOverflow=off  InputSameDT=off
  EZECal : Outport  VectorParamsAs1DForOutWhenUnconnected=off
  wires:
  Switch/1 -> EZECal/1
  FirstStepPassFlg/1 -> Switch/2
  Cal2/1 -> Switch/1
  Cal1/1 -> Switch/3

== system SecRwLtStCalib/SecRwLtStBkReclnTrgtPosSelc_1_Cal_sys/Subsystem1/Subsystem3 ==
  FirstStepPassFlg : Inport
  Cal2 : Inport  Port=2
  Cal1 : Inport  Port=3
  Switch : Switch  Criteria=u2 > Threshold  SaturateOnIntegerOverflow=off  InputSameDT=off
  EZECal : Outport  VectorParamsAs1DForOutWhenUnconnected=off
  wires:
  Cal1/1 -> Switch/3
  Cal2/1 -> Switch/1
  FirstStepPassFlg/1 -> Switch/2
  Switch/1 -> EZECal/1

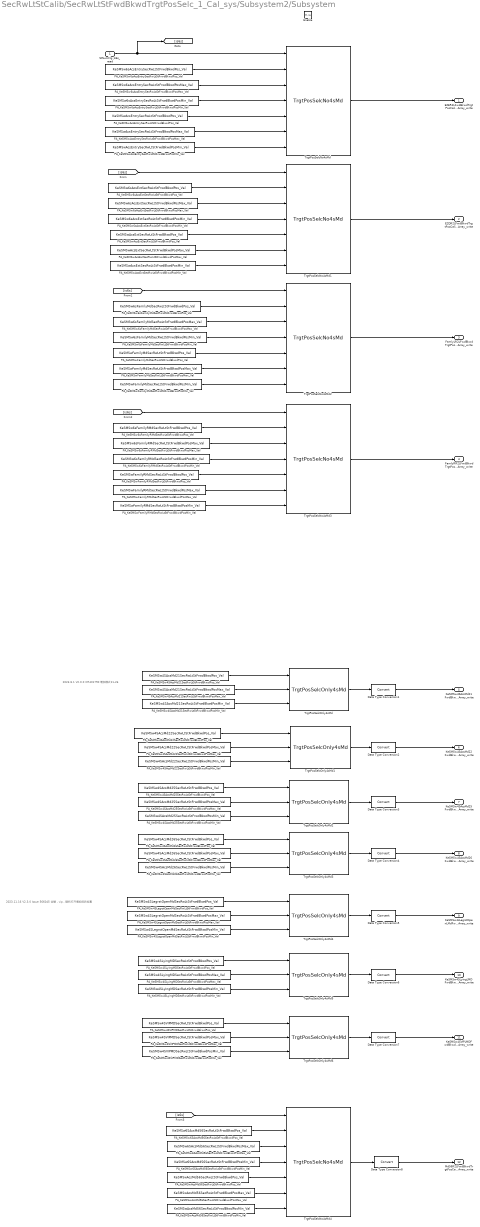
== system SecRwLtStCalib/SecRwLtStFwdBkwdTrgtPosSelc_1_Cal_sys/Subsystem2/Subsystem ==
  note: 2023.11.16 V2.3.0 Issue 566045 全躺，vip，腿托打开增加前后位置
  note: 2023.8.1 V2.0.0 CR401790 增加模式21-26
  StNumFlg_Is6s_read : Inport
  Enable : EnablePort
  Data Type Conversion{1..8} (8 alike) : DataTypeConversion  SaturateOnIntegerOverflow=off  RndMeth=Floor
  PA_KeSMSw4SAcsMd21SecRwLtStFrwdBkwdPosMax_Val : Constant  Value=KeSMSw4SAcsMd21SecRwLtStFrwdBkwdPosMax_Val
  PA_KeSMSw4SAcsMd21SecRwLtStFrwdBkwdPosMin_Val : Constant  Value=KeSMSw4SAcsMd21SecRwLtStFrwdBkwdPosMin_Val
  PA_KeSMSw4SAcsMd21SecRwLtStFrwdBkwdPos_Val : Constant  Value=KeSMSw4SAcsMd21SecRwLtStFrwdBkwdPos_Val
  PA_KeSMSw4SAcsMd22SecRwLtStFrwdBkwdPosMax_Val : Constant  Value=KeSMSw4SAcsMd22SecRwLtStFrwdBkwdPosMax_Val
  PA_KeSMSw4SAcsMd22SecRwLtStFrwdBkwdPosMin_Val : Constant  Value=KeSMSw4SAcsMd22SecRwLtStFrwdBkwdPosMin_Val
  PA_KeSMSw4SAcsMd22SecRwLtStFrwdBkwdPos_Val : Constant  Value=KeSMSw4SAcsMd22SecRwLtStFrwdBkwdPos_Val
  PA_KeSMSw4SAcsMd25SecRwLtStFrwdBkwdPosMax_Val : Constant  Value=KeSMSw4SAcsMd25SecRwLtStFrwdBkwdPosMax_Val
  PA_KeSMSw4SAcsMd25SecRwLtStFrwdBkwdPosMin_Val : Constant  Value=KeSMSw4SAcsMd25SecRwLtStFrwdBkwdPosMin_Val
  PA_KeSMSw4SAcsMd25SecRwLtStFrwdBkwdPos_Val : Constant  Value=KeSMSw4SAcsMd25SecRwLtStFrwdBkwdPos_Val
  PA_KeSMSw4SAcsMd26SecRwLtStFrwdBkwdPosMax_Val : Constant  Value=KeSMSw4SAcsMd26SecRwLtStFrwdBkwdPosMax_Val
  PA_KeSMSw4SAcsMd26SecRwLtStFrwdBkwdPosMin_Val : Constant  Value=KeSMSw4SAcsMd26SecRwLtStFrwdBkwdPosMin_Val
  PA_KeSMSw4SAcsMd26SecRwLtStFrwdBkwdPos_Val : Constant  Value=KeSMSw4SAcsMd26SecRwLtStFrwdBkwdPos_Val
  PA_KeSMSw4SLegrstOpenMdSecRwLtStFrwdBkwdPosMax_Val : Constant  Value=KeSMSw4SLegrstOpenMdSecRwLtStFrwdBkwdPosMax_Val
  PA_KeSMSw4SLegrstOpenMdSecRwLtStFrwdBkwdPosMin_Val : Constant  Value=KeSMSw4SLegrstOpenMdSecRwLtStFrwdBkwdPosMin_Val
  PA_KeSMSw4SLegrstOpenMdSecRwLtStFrwdBkwdPos_Val : Constant  Value=KeSMSw4SLegrstOpenMdSecRwLtStFrwdBkwdPos_Val
  PA_KeSMSw4SLyingMDSecRwLtStFrwdBkwdPosMax_Val : Constant  Value=KeSMSw4SLyingMDSecRwLtStFrwdBkwdPosMax_Val
  PA_KeSMSw4SLyingMDSecRwLtStFrwdBkwdPosMin_Val : Constant  Value=KeSMSw4SLyingMDSecRwLtStFrwdBkwdPosMin_Val
  PA_KeSMSw4SLyingMDSecRwLtStFrwdBkwdPos_Val : Constant  Value=KeSMSw4SLyingMDSecRwLtStFrwdBkwdPos_Val
  PA_KeSMSw4SVIPMDSecRwLtStFrwdBkwdPosMax_Val : Constant  Value=KeSMSw4SVIPMDSecRwLtStFrwdBkwdPosMax_Val
  PA_KeSMSw4SVIPMDSecRwLtStFrwdBkwdPosMin_Val : Constant  Value=KeSMSw4SVIPMDSecRwLtStFrwdBkwdPosMin_Val
  PA_KeSMSw4SVIPMDSecRwLtStFrwdBkwdPos_Val : Constant  Value=KeSMSw4SVIPMDSecRwLtStFrwdBkwdPos_Val
  PA_KeSMSw6SAcsMd56SecRwLtStFrwdBkwdPosMax_Val : Constant  Value=KeSMSw6SAcsMd56SecRwLtStFrwdBkwdPosMax_Val
  PA_KeSMSw6SAcsMd56SecRwLtStFrwdBkwdPosMin_Val : Constant  Value=KeSMSw6SAcsMd56SecRwLtStFrwdBkwdPosMin_Val
  PA_KeSMSw6SAcsMd56SecRwLtStFrwdBkwdPos_Val : Constant  Value=KeSMSw6SAcsMd56SecRwLtStFrwdBkwdPos_Val
  PA_KeSMSw6sAcsEntrySecRwLtStFrwdBkwdPosMax_Val : Constant  Value=KeSMSw6sAcsEntrySecRwLtStFrwdBkwdPosMax_Val
  PA_KeSMSw6sAcsEntrySecRwLtStFrwdBkwdPosMin_Val : Constant  Value=KeSMSw6sAcsEntrySecRwLtStFrwdBkwdPosMin_Val
  PA_KeSMSw6sAcsEntrySecRwLtStFrwdBkwdPos_Val : Constant  Value=KeSMSw6sAcsEntrySecRwLtStFrwdBkwdPos_Val
  PA_KeSMSw6sAcsExtSecRwLtStFrwdBkwdPosMax_Val : Constant  Value=KeSMSw6sAcsExtSecRwLtStFrwdBkwdPosMax_Val
  PA_KeSMSw6sAcsExtSecRwLtStFrwdBkwdPosMin_Val : Constant  Value=KeSMSw6sAcsExtSecRwLtStFrwdBkwdPosMin_Val
  PA_KeSMSw6sAcsExtSecRwLtStFrwdBkwdPos_Val : Constant  Value=KeSMSw6sAcsExtSecRwLtStFrwdBkwdPos_Val
  PA_KeSMSw6sFamilyMdSecRwLtStFrwdBkwdPosMax_Val : Constant  Value=KeSMSw6sFamilyMdSecRwLtStFrwdBkwdPosMax_Val
  PA_KeSMSw6sFamilyMdSecRwLtStFrwdBkwdPosMin_Val : Constant  Value=KeSMSw6sFamilyMdSecRwLtStFrwdBkwdPosMin_Val
  PA_KeSMSw6sFamilyMdSecRwLtStFrwdBkwdPos_Val : Constant  Value=KeSMSw6sFamilyMdSecRwLtStFrwdBkwdPos_Val
  PA_KeSMSw6sFamilyRMdSecRwLtStFrwdBkwdPosMax_Val : Constant  Value=KeSMSw6sFamilyRMdSecRwLtStFrwdBkwdPosMax_Val
  PA_KeSMSw6sFamilyRMdSecRwLtStFrwdBkwdPosMin_Val : Constant  Value=KeSMSw6sFamilyRMdSecRwLtStFrwdBkwdPosMin_Val
  PA_KeSMSw6sFamilyRMdSecRwLtStFrwdBkwdPos_Val : Constant  Value=KeSMSw6sFamilyRMdSecRwLtStFrwdBkwdPos_Val
  PA_KeSMSwAcsEntrySecRwLtStFrwdBkwdPosMax_Val : Constant  Value=KeSMSwAcsEntrySecRwLtStFrwdBkwdPosMax_Val
  PA_KeSMSwAcsEntrySecRwLtStFrwdBkwdPosMin_Val : Constant  Value=KeSMSwAcsEntrySecRwLtStFrwdBkwdPosMin_Val
  PA_KeSMSwAcsEntrySecRwLtStFrwdBkwdPos_Val : Constant  Value=KeSMSwAcsEntrySecRwLtStFrwdBkwdPos_Val
  PA_KeSMSwAcsExtSecRwLtStFrwdBkwdPosMax_Val : Constant  Value=KeSMSwAcsExtSecRwLtStFrwdBkwdPosMax_Val
  PA_KeSMSwAcsExtSecRwLtStFrwdBkwdPosMin_Val : Constant  Value=KeSMSwAcsExtSecRwLtStFrwdBkwdPosMin_Val
  PA_KeSMSwAcsExtSecRwLtStFrwdBkwdPos_Val : Constant  Value=KeSMSwAcsExtSecRwLtStFrwdBkwdPos_Val
  PA_KeSMSwAcsMd56SecRwLtStFrwdBkwdPosMax_Val : Constant  Value=KeSMSwAcsMd56SecRwLtStFrwdBkwdPosMax_Val
  PA_KeSMSwAcsMd56SecRwLtStFrwdBkwdPosMin_Val : Constant  Value=KeSMSwAcsMd56SecRwLtStFrwdBkwdPosMin_Val
  PA_KeSMSwAcsMd56SecRwLtStFrwdBkwdPos_Val : Constant  Value=KeSMSwAcsMd56SecRwLtStFrwdBkwdPos_Val
  PA_KeSMSwFamilyMdSecRwLtStFrwdBkwdPosMax_Val : Constant  Value=KeSMSwFamilyMdSecRwLtStFrwdBkwdPosMax_Val
  PA_KeSMSwFamilyMdSecRwLtStFrwdBkwdPosMin_Val : Constant  Value=KeSMSwFamilyMdSecRwLtStFrwdBkwdPosMin_Val
  PA_KeSMSwFamilyMdSecRwLtStFrwdBkwdPos_Val : Constant  Value=KeSMSwFamilyMdSecRwLtStFrwdBkwdPos_Val
  PA_KeSMSwFamilyRMdSecRwLtStFrwdBkwdPosMax_Val : Constant  Value=KeSMSwFamilyRMdSecRwLtStFrwdBkwdPosMax_Val
  PA_KeSMSwFamilyRMdSecRwLtStFrwdBkwdPosMin_Val : Constant  Value=KeSMSwFamilyRMdSecRwLtStFrwdBkwdPosMin_Val
  PA_KeSMSwFamilyRMdSecRwLtStFrwdBkwdPos_Val : Constant  Value=KeSMSwFamilyRMdSecRwLtStFrwdBkwdPos_Val
  TrgtPosSelcNo4sMd{,1..4} (5 alike) : TrgtPosSelcLib/TrgtPosSelcNo4sMd  SystemSampleTime=-1  VariantActivationTime=update diagram  AllowFlexibleInterface=on  Latency=0  AutoFrameSizeCalculation=off
  TrgtPosSelcOnly4sMd{,1..6} (7 alike) : TrgtPosSelcLib/TrgtPosSelcOnly4sMd  SystemSampleTime=-1  VariantActivationTime=update diagram  AllowFlexibleInterface=on  Latency=0  AutoFrameSizeCalculation=off
  EZER2LFwdBkwdTrgtPosCalib_TrgtPosArray_write : Outport  VectorParamsAs1DForOutWhenUnconnected=off
      settings: EnsureOutportIsVirtual=on
  EZQR2LFwdBkwdTrgtPosCalib_TrgtPosArray_write : Outport  Port=2  VectorParamsAs1DForOutWhenUnconnected=off
      settings: EnsureOutportIsVirtual=on
  FamlyLR2LFwdBkwdTrgtPosCalib_TrgtPosArray_write : Outport  Port=3  VectorParamsAs1DForOutWhenUnconnected=off
      settings: EnsureOutportIsVirtual=on
  FamlyRR2LFwdBkwdTrgtPosCalib_TrgtPosArray_write : Outport  Port=4  VectorParamsAs1DForOutWhenUnconnected=off
      settings: EnsureOutportIsVirtual=on
  KeSMSw4SAcsMd21FwdBkwdTrgtPosCalib_TrgtPosArray_write : Outport  Port=5  VectorParamsAs1DForOutWhenUnconnected=off
      settings: EnsureOutportIsVirtual=on
  KeSMSw4SAcsMd22FwdBkwdTrgtPosCalib_TrgtPosArray_write : Outport  Port=6  VectorParamsAs1DForOutWhenUnconnected=off
      settings: EnsureOutportIsVirtual=on
  KeSMSw4SAcsMd25FwdBkwdTrgtPosCalib_TrgtPosArray_write : Outport  Port=7  VectorParamsAs1DForOutWhenUnconnected=off
      settings: EnsureOutportIsVirtual=on
  KeSMSw4SAcsMd26FwdBkwdTrgtPosCalib_TrgtPosArray_write : Outport  Port=8  VectorParamsAs1DForOutWhenUnconnected=off
      settings: EnsureOutportIsVirtual=on
  KeSMSw4sLegrstOpenLMdFwdBkwdTrgtPosCalib_TrgtPosArray_write : Outport  Port=9  VectorParamsAs1DForOutWhenUnconnected=off
      settings: EnsureOutportIsVirtual=on
  KeSMSw4SLyingLMDFwdBkwdTrgtPosCalib_TrgtPosArray_write : Outport  Port=10  VectorParamsAs1DForOutWhenUnconnected=off
      settings: EnsureOutportIsVirtual=on
  KeSMSw4SVIPLMDFwdBkwdTrgtPosCalib_TrgtPosArray_write : Outport  Port=11  VectorParamsAs1DForOutWhenUnconnected=off
      settings: EnsureOutportIsVirtual=on
  Md56R2LFwdBkwdTrgtPosCalib_TrgtPosArray_write : Outport  Port=12  VectorParamsAs1DForOutWhenUnconnected=off
      settings: EnsureOutportIsVirtual=on
  wires:
  TrgtPosSelcNo4sMd1/1 -> EZQR2LFwdBkwdTrgtPosCalib_TrgtPosArray_write/1
  TrgtPosSelcNo4sMd3/1 -> FamlyRR2LFwdBkwdTrgtPosCalib_TrgtPosArray_write/1
  TrgtPosSelcNo4sMd/1 -> EZER2LFwdBkwdTrgtPosCalib_TrgtPosArray_write/1
  TrgtPosSelcNo4sMd2/1 -> FamlyLR2LFwdBkwdTrgtPosCalib_TrgtPosArray_write/1
  StNumFlg_Is6s_read/1 -> [is6s], TrgtPosSelcNo4sMd/1
  PA_KeSMSw6sAcsEntrySecRwLtStFrwdBkwdPos_Val/1 -> TrgtPosSelcNo4sMd/2
  PA_KeSMSw6sAcsEntrySecRwLtStFrwdBkwdPosMax_Val/1 -> TrgtPosSelcNo4sMd/3
  PA_KeSMSw6sAcsEntrySecRwLtStFrwdBkwdPosMin_Val/1 -> TrgtPosSelcNo4sMd/4
  PA_KeSMSw6sAcsExtSecRwLtStFrwdBkwdPosMin_Val/1 -> TrgtPosSelcNo4sMd1/4
  PA_KeSMSw6sAcsExtSecRwLtStFrwdBkwdPosMax_Val/1 -> TrgtPosSelcNo4sMd1/3
  PA_KeSMSw6sAcsExtSecRwLtStFrwdBkwdPos_Val/1 -> TrgtPosSelcNo4sMd1/2
  PA_KeSMSw6sFamilyMdSecRwLtStFrwdBkwdPos_Val/1 -> TrgtPosSelcNo4sMd2/2
  PA_KeSMSw6sFamilyMdSecRwLtStFrwdBkwdPosMax_Val/1 -> TrgtPosSelcNo4sMd2/3
  PA_KeSMSw6sFamilyMdSecRwLtStFrwdBkwdPosMin_Val/1 -> TrgtPosSelcNo4sMd2/4
  PA_KeSMSw6sFamilyRMdSecRwLtStFrwdBkwdPosMin_Val/1 -> TrgtPosSelcNo4sMd3/4
  PA_KeSMSw6sFamilyRMdSecRwLtStFrwdBkwdPosMax_Val/1 -> TrgtPosSelcNo4sMd3/3
  PA_KeSMSw6sFamilyRMdSecRwLtStFrwdBkwdPos_Val/1 -> TrgtPosSelcNo4sMd3/2
  PA_KeSMSwAcsEntrySecRwLtStFrwdBkwdPos_Val/1 -> TrgtPosSelcNo4sMd/5
  PA_KeSMSwAcsEntrySecRwLtStFrwdBkwdPosMax_Val/1 -> TrgtPosSelcNo4sMd/6
  PA_KeSMSwAcsEntrySecRwLtStFrwdBkwdPosMin_Val/1 -> TrgtPosSelcNo4sMd/7
  PA_KeSMSwAcsExtSecRwLtStFrwdBkwdPos_Val/1 -> TrgtPosSelcNo4sMd1/5
  PA_KeSMSwAcsExtSecRwLtStFrwdBkwdPosMax_Val/1 -> TrgtPosSelcNo4sMd1/6
  PA_KeSMSwAcsExtSecRwLtStFrwdBkwdPosMin_Val/1 -> TrgtPosSelcNo4sMd1/7
  PA_KeSMSwFamilyMdSecRwLtStFrwdBkwdPosMin_Val/1 -> TrgtPosSelcNo4sMd2/7
  PA_KeSMSwFamilyMdSecRwLtStFrwdBkwdPosMax_Val/1 -> TrgtPosSelcNo4sMd2/6
  PA_KeSMSwFamilyMdSecRwLtStFrwdBkwdPos_Val/1 -> TrgtPosSelcNo4sMd2/5
  PA_KeSMSwFamilyRMdSecRwLtStFrwdBkwdPos_Val/1 -> TrgtPosSelcNo4sMd3/5
  PA_KeSMSwFamilyRMdSecRwLtStFrwdBkwdPosMax_Val/1 -> TrgtPosSelcNo4sMd3/6
  PA_KeSMSwFamilyRMdSecRwLtStFrwdBkwdPosMin_Val/1 -> TrgtPosSelcNo4sMd3/7
  [is6s] -> TrgtPosSelcNo4sMd1/1
  [is6s] -> TrgtPosSelcNo4sMd2/1
  [is6s] -> TrgtPosSelcNo4sMd3/1
  TrgtPosSelcOnly4sMd/1 -> Data Type Conversion1/1
  TrgtPosSelcOnly4sMd3/1 -> Data Type Conversion4/1
  TrgtPosSelcOnly4sMd2/1 -> Data Type Conversion3/1
  TrgtPosSelcOnly4sMd1/1 -> Data Type Conversion2/1
  PA_KeSMSw4SAcsMd26SecRwLtStFrwdBkwdPosMax_Val/1 -> TrgtPosSelcOnly4sMd3/2
  PA_KeSMSw4SAcsMd26SecRwLtStFrwdBkwdPosMin_Val/1 -> TrgtPosSelcOnly4sMd3/3
  PA_KeSMSw4SAcsMd26SecRwLtStFrwdBkwdPos_Val/1 -> TrgtPosSelcOnly4sMd3/1
  PA_KeSMSw4SAcsMd25SecRwLtStFrwdBkwdPosMax_Val/1 -> TrgtPosSelcOnly4sMd2/2
  PA_KeSMSw4SAcsMd25SecRwLtStFrwdBkwdPosMin_Val/1 -> TrgtPosSelcOnly4sMd2/3
  PA_KeSMSw4SAcsMd25SecRwLtStFrwdBkwdPos_Val/1 -> TrgtPosSelcOnly4sMd2/1
  PA_KeSMSw4SAcsMd22SecRwLtStFrwdBkwdPosMax_Val/1 -> TrgtPosSelcOnly4sMd1/2
  PA_KeSMSw4SAcsMd22SecRwLtStFrwdBkwdPosMin_Val/1 -> TrgtPosSelcOnly4sMd1/3
  PA_KeSMSw4SAcsMd22SecRwLtStFrwdBkwdPos_Val/1 -> TrgtPosSelcOnly4sMd1/1
  PA_KeSMSw4SAcsMd21SecRwLtStFrwdBkwdPosMax_Val/1 -> TrgtPosSelcOnly4sMd/2
  PA_KeSMSw4SAcsMd21SecRwLtStFrwdBkwdPosMin_Val/1 -> TrgtPosSelcOnly4sMd/3
  PA_KeSMSw4SAcsMd21SecRwLtStFrwdBkwdPos_Val/1 -> TrgtPosSelcOnly4sMd/1
  Data Type Conversion1/1 -> KeSMSw4SAcsMd21FwdBkwdTrgtPosCalib_TrgtPosArray_write/1
  Data Type Conversion2/1 -> KeSMSw4SAcsMd22FwdBkwdTrgtPosCalib_TrgtPosArray_write/1
  Data Type Conversion3/1 -> KeSMSw4SAcsMd25FwdBkwdTrgtPosCalib_TrgtPosArray_write/1
  Data Type Conversion4/1 -> KeSMSw4SAcsMd26FwdBkwdTrgtPosCalib_TrgtPosArray_write/1
  PA_KeSMSw4SLegrstOpenMdSecRwLtStFrwdBkwdPos_Val/1 -> TrgtPosSelcOnly4sMd4/1
  PA_KeSMSw4SLegrstOpenMdSecRwLtStFrwdBkwdPosMin_Val/1 -> TrgtPosSelcOnly4sMd4/3
  PA_KeSMSw4SLegrstOpenMdSecRwLtStFrwdBkwdPosMax_Val/1 -> TrgtPosSelcOnly4sMd4/2
  TrgtPosSelcOnly4sMd4/1 -> Data Type Conversion5/1
  TrgtPosSelcOnly4sMd5/1 -> Data Type Conversion6/1
  PA_KeSMSw4SLyingMDSecRwLtStFrwdBkwdPosMax_Val/1 -> TrgtPosSelcOnly4sMd5/2
  PA_KeSMSw4SLyingMDSecRwLtStFrwdBkwdPosMin_Val/1 -> TrgtPosSelcOnly4sMd5/3
  PA_KeSMSw4SLyingMDSecRwLtStFrwdBkwdPos_Val/1 -> TrgtPosSelcOnly4sMd5/1
  PA_KeSMSw4SVIPMDSecRwLtStFrwdBkwdPos_Val/1 -> TrgtPosSelcOnly4sMd6/1
  PA_KeSMSw4SVIPMDSecRwLtStFrwdBkwdPosMin_Val/1 -> TrgtPosSelcOnly4sMd6/3
  PA_KeSMSw4SVIPMDSecRwLtStFrwdBkwdPosMax_Val/1 -> TrgtPosSelcOnly4sMd6/2
  TrgtPosSelcOnly4sMd6/1 -> Data Type Conversion7/1
  Data Type Conversion7/1 -> KeSMSw4SVIPLMDFwdBkwdTrgtPosCalib_TrgtPosArray_write/1
  Data Type Conversion5/1 -> KeSMSw4sLegrstOpenLMdFwdBkwdTrgtPosCalib_TrgtPosArray_write/1
  Data Type Conversion6/1 -> KeSMSw4SLyingLMDFwdBkwdTrgtPosCalib_TrgtPosArray_write/1
  [is6s] -> TrgtPosSelcNo4sMd4/1
  PA_KeSMSw6SAcsMd56SecRwLtStFrwdBkwdPos_Val/1 -> TrgtPosSelcNo4sMd4/2
  PA_KeSMSw6SAcsMd56SecRwLtStFrwdBkwdPosMax_Val/1 -> TrgtPosSelcNo4sMd4/3
  PA_KeSMSwAcsMd56SecRwLtStFrwdBkwdPosMin_Val/1 -> TrgtPosSelcNo4sMd4/7
  PA_KeSMSwAcsMd56SecRwLtStFrwdBkwdPosMax_Val/1 -> TrgtPosSelcNo4sMd4/6
  PA_KeSMSwAcsMd56SecRwLtStFrwdBkwdPos_Val/1 -> TrgtPosSelcNo4sMd4/5
  PA_KeSMSw6SAcsMd56SecRwLtStFrwdBkwdPosMin_Val/1 -> TrgtPosSelcNo4sMd4/4
  TrgtPosSelcNo4sMd4/1 -> Data Type Conversion8/1
  Data Type Conversion8/1 -> Md56R2LFwdBkwdTrgtPosCalib_TrgtPosArray_write/1

== system SecRwLtStCalib/SecRwLtStFwdBkwdTrgtPosSelc_1_Cal_sys/Subsystem2/Subsystem1 ==
  IfVeSMSuSecRwRtStFrwdBkwdPos_Val_read : Inport
  IfVeSMSuSecRwRtStFrwdBkwdPosV_Val_read : Inport  Port=2
  Constant : Constant  Value=0  OutDataTypeStr=uint16
  NOT : Logic  Operator=NOT  AllPortsSameDT=off  OutDataTypeStr=boolean
  Switch : Switch  Criteria=u2 > Threshold  SaturateOnIntegerOverflow=off  InputSameDT=off
  TrgtPos : Outport  VectorParamsAs1DForOutWhenUnconnected=off
  wires:
  IfVeSMSuSecRwRtStFrwdBkwdPosV_Val_read/1 -> NOT/1
  Constant/1 -> Switch/3
  IfVeSMSuSecRwRtStFrwdBkwdPos_Val_read/1 -> Switch/1
  NOT/1 -> Switch/2
  Switch/1 -> TrgtPos/1
